simulink model "L58"  (Simulink 8.0)
settings: Solver=ode45  SolverMode=SingleTasking  StartTime=0.0  StopTime=50  RelTol=1e-3
settings Model: Creator=mebuffet  LastModifiedBy=mebuffet  CovMetricSettings=dwe  CovHtmlReporting=off  covSaveCumulativeToWorkspaceVar=off  CovSaveSingleToWorkspaceVar=off  CovExternalEMLEnable=on
settings DataIOCC: LimitDataPoints=off  SaveFormat=StructureWithTime
settings OptimizationCC: ExpressionDepthLimit=128
settings DebuggingCC: UnderspecifiedInitializationDetection=Simplified  MergeDetectMultiDrivingBlocksExec=error  SolverPrmCheckMsg=none  FrameProcessingCompatibilityMsg=error  StateNameClashWarn=none  SFUnexpectedBacktrackingDiag=error  SFNoUnconditionalDefaultTransitionDiag=error
settings HardwareCC: ProdBitPerPointer=64  ProdLargestAtomicFloat=Float  ProdIntDivRoundTo=Zero  ProdEndianess=LittleEndian  ProdHWDeviceType=Specified
settings ModelReferenceCC: PropagateSignalLabelsOutOfModel=on
settings CodeAppCC: CustomSymbolStrType=$N$R$M_T
settings GRTTargetCC: CodeReplacementLibrary=C99 (ISO)  GeneratePreprocessorConditionals=Use local settings

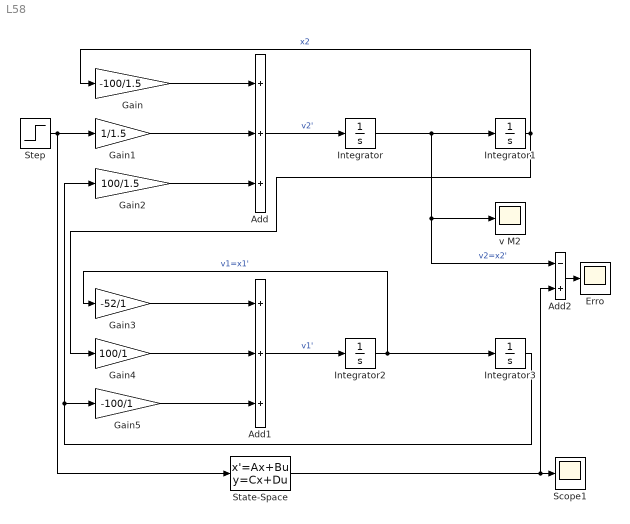
== system L58 ==
  Add : Sum  Inputs=+++
  Add1 : Sum  Inputs=+++
  Add2 : Sum  Inputs=-+
  Erro : Scope
      settings: TimeRange=auto  MaxDataPoints=5000  SaveToWorkspace=off  SaveName=ScopeData2  YMin=-0.00000000000000015  YMax=0.00000000000000029  SampleTime=-1
  Gain : Gain  Gain=-100/1.5
  Gain1 : Gain  Gain=1/1.5
  Gain2 : Gain  Gain=100/1.5
  Gain3 : Gain  Gain=-52/1
  Gain4 : Gain  Gain=100/1
  Gain5 : Gain  Gain=-100/1
  Integrator{,1..3} (4 alike) : Integrator
  Scope1 : Scope
      settings: TimeRange=auto  MaxDataPoints=5000  SaveToWorkspace=off  YMin=-0.09627  YMax=0.10479  SampleTime=-1
  State-Space : StateSpace  A=[0 1 0 0; -100/1 -52/1 100/1 0; 0 0 0 1; 100/1.5 0 -100/1.5 0]  B=[0; 0; 0; 1/1.5]  C=[0 0 0 1]  D=0  X0=0
  Step : Step  Before=1  After=0  SampleTime=0
  v M2 : Scope
      settings: TimeRange=auto  MaxDataPoints=5000  SaveToWorkspace=off  SaveName=ScopeData  YMin=-0.09621  YMax=0.10488  SampleTime=-1
  wires:
  Gain2/1 -> Add/3
  Gain1/1 -> Add/2
  Gain/1 -> Add/1
  Step/1 -> Gain1/1, State-Space/1
  Add/1 -> Integrator/1  "v2'"
  Integrator/1 -> v M2/1, Add2/1, Integrator1/1  "v2=x2'"
  Gain5/1 -> Add1/3
  Gain4/1 -> Add1/2
  Gain3/1 -> Add1/1
  Add1/1 -> Integrator2/1  "v1'"
  Integrator2/1 -> Integrator3/1, Gain3/1  "v1=x1'"
  State-Space/1 -> Scope1/1, Add2/2
  Add2/1 -> Erro/1
  Integrator1/1 -> Gain4/1, Gain/1  "x2"
  Integrator3/1 -> Gain5/1, Gain2/1
